simulink model "LinearStateSpaceModelLQRReferenceFollowing"  (R2014b)
settings: Solver=ode45  StartTime=0.0  StopTime=60  RelTol=1e-6
undefined symbols (not defined in the file): linearized_state_space_model, lqr_gain, N_reference
libraries: simulink x1
settings Model: Creator=NagyZe  LastModifiedBy=NagyZe

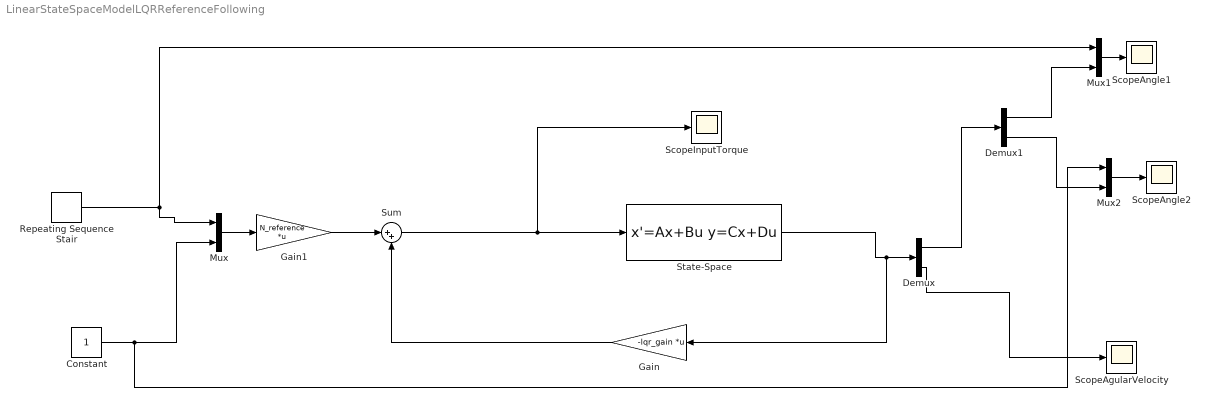
== system LinearStateSpaceModelLQRReferenceFollowing ==
  Constant : Constant
  Demux : Demux  Outputs=2
  Demux1 : Demux  Outputs=2
  Gain : Gain  Gain=-lqr_gain  Multiplication=Matrix(K*u) (u vector)
  Gain1 : Gain  Gain=N_reference  Multiplication=Matrix(K*u) (u vector)
  Mux : Mux  Inputs=2
  Mux1 : Mux  Inputs=2
  Mux2 : Mux  Inputs=2
  Repeating Sequence Stair : simulink/Sources/Repeating Sequence Stair  OutValues=[1 4 6 2 0].'  tsamp=5  OutMin=[]  OutMax=[]  OutDataTypeStr=double  OutputDataTypeScalingMode=double  OutDataType=fixdt(0,8)  ConRadixGroup=Best Precision: Vector-wise  OutScaling=2^-12
  ScopeAgularVelocity : Scope
      settings: TimeRange=10  YMin=-40  YMax=30  SaveName=jointVelocity
  ScopeAngle1 : Scope
      settings: TimeRange=10  YMin=-0.005  YMax=0.03  SaveName=jointAngle
  ScopeAngle2 : Scope
      settings: TimeRange=10  YMin=-0.005  YMax=0.03  SaveName=jointAngle1
  ScopeInputTorque : Scope
      settings: YMin=-1  YMax=1  SaveName=torque
  State-Space : StateSpace  A=linearized_state_space_model.A  B=linearized_state_space_model.B  C=eye(4)  D=zeros(4,2)  X0=[0.2 0.1 0 0]
  Sum : Sum  Inputs=|++
  wires:
  State-Space/1 -> Gain/1, Demux/1
  Demux/2 -> ScopeAgularVelocity/1
  Gain1/1 -> Sum/1
  Repeating Sequence Stair/1 -> Mux/1, Mux1/1
  Mux/1 -> Gain1/1
  Constant/1 -> Mux2/1, Mux/2
  Gain/1 -> Sum/2
  Sum/1 -> ScopeInputTorque/1, State-Space/1
  Demux/1 -> Demux1/1
  Demux1/1 -> Mux1/2
  Mux1/1 -> ScopeAngle1/1
  Mux2/1 -> ScopeAngle2/1
  Demux1/2 -> Mux2/2
